simulink model "ProyectoDeControl"  (Simulink 10.1)
settings: Solver=ode45  StartTime=0.0  StopTime=inf  RelTol=1e-3  EnableMultiTasking=on
undefined symbols (not defined in the file or in its folder): serial
libraries: instrumentlib x3, simulink x1
settings Model: Creator=Jorge  LastModifiedBy=Jeremias
settings DataIOCC: LimitDataPoints=on  SignalLoggingSaveFormat=ModelDataLogs
settings OptimizationCC: ExpressionDepthLimit=2147483647
settings DebuggingCC: SolverPrmCheckMsg=warning  FcnCallInpInsideContextMsg=warning  StateNameClashWarn=warning

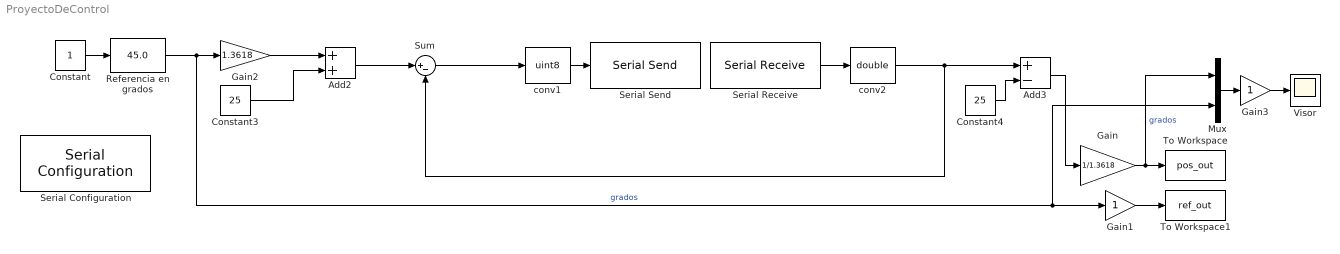
== system ProyectoDeControl ==
  Add2 : Sum
  Add3 : Sum  Inputs=+-
  Constant : Constant  SampleTime=0.02
  Constant3 : Constant  Value=25  SampleTime=0.02
  Constant4 : Constant  Value=25  SampleTime=0.02
  Gain : Gain  Gain=1/1.3618
  Gain1 : Gain
  Gain2 : Gain  Gain=1.3618
  Gain3 : Gain
  Mux : Mux  Inputs=2
  Referencia en grados : simulink/Math Operations/Slider Gain  gain=45.0  low=0  high=60
  Serial Configuration : instrumentlib/Serial Configuration  Priority=-200000  ComPortMenu=<Please select a port...>  ComPort=COM4  ObjConstructor=serial('COM4');  BaudRate=9600  DataBits=8  Parity=none  StopBits=1  FlowControl=none  Timeout=10  ByteOrder=LittleEndian
  Serial Receive : instrumentlib/Serial Receive  ComPortMenu=<Please select a port...>  ComPort=COM4  ObjConstructor=serial('COM4');  Terminator=<none>  DataSize=[1 1]  DataType=uint8  EnableBlockingMode=on  ActionDataUnavailable=Output last received value  CustomValue=0  SampleTime=0.01
  Serial Send : instrumentlib/Serial Send  ComPortMenu=<Please select a port...>  ComPort=COM4  ObjConstructor=serial('COM4');  Terminator=<none>  EnableBlockingMode=on
  Sum : Sum  Inputs=|+-
  To Workspace : ToWorkspace  VariableName=pos_out  SampleTime=-1
  To Workspace1 : ToWorkspace  VariableName=ref_out  SampleTime=-1
  Visor : Scope
  conv1 : DataTypeConversion  OutDataTypeStr=uint8  SampleTime=0.01
  conv2 : DataTypeConversion  OutDataTypeStr=double
  wires:
  conv1/1 -> Serial Send/1
  Serial Receive/1 -> conv2/1
  Constant/1 -> Referencia en grados/1
  Gain1/1 -> To Workspace1/1
  Mux/1 -> Gain3/1
  Gain3/1 -> Visor/1
  Gain2/1 -> Add2/1
  Referencia en grados/1 -> Mux/2, Gain1/1, Gain2/1  "grados"
  Constant3/1 -> Add2/2
  Constant4/1 -> Add3/2
  Add3/1 -> Gain/1
  Gain/1 -> To Workspace/1, Mux/1  "grados"
  Add2/1 -> Sum/1
  Sum/1 -> conv1/1
  conv2/1 -> Sum/2, Add3/1
